simulink model "Demo_CooperativeDriving_cs"  (Simulink 7.6)
settings: Solver=ode5  SolverMode=SingleTasking  StartTime=0.0  StopTime=8  FixedStep=1/20  RelTol=1e-3
PreLoadFcn:
  | check_NUTS_defined
  | model_closed = 0;
  | assignin('base',['model_closed_' bdroot],false);
InitFcn:
  | PreScanExperimentInitFcn(bdroot)
StopFcn:
  | PreScanExperimentStopFcn(bdroot);
  | 
values from neighbouring files (symbols this model uses):
  Cf = (MLV+MRV)*g/2    (= 5460.246)    [shared_pars.m]
  Cr = (MLA+MRA)*g/2    (= 3937.734)    [shared_pars.m]
  Jzz = J_zz + 2*m_wheel*lva^2 + 2*m_wheel*laa^2    (= 3255.36268364)    [shared_pars.m]
  Kaa = 200000    [shared_pars.m]
  Kf = Kva/(g*(MLV+MRV))    (= 18.3141931701)    [shared_pars.m]
  Kr = Kaa/(g*(MLA+MRA))    (= 25.3953161895)    [shared_pars.m]
  Kva = 200000    [shared_pars.m]
  laa = l - lva    (= 1.67328601253)    [shared_pars.m]
  lva = l*(MLA+MRA)/m    (= 1.20671398747)    [shared_pars.m]
  m = MLV+MRV+MLA+MRA    (= 1916)    [shared_pars.m]
  Mu = 1    [simulinkmodel.m]
  relax_on = 0    [simulinkmodel.m]
  sigma_f = 0.65    [simulinkmodel.m]
  sigma_r = 0.65    [simulinkmodel.m]
  TyreType = 1    [simulinkmodel.m]
undefined symbols (not defined in the file or in its folder): DiscIntNeverNeededParam
libraries: PreScanSimulinkLibrary x14, PreScanUsefulBlocks x6, simulink_extras x5
(part 4 of 6)

== system Demo_CooperativeDriving_cs/Citroen_C3_1/Swarm Behavior/Polar2Cart1 ==
  R : Inport
  theta : Inport  Port=2
  Degrees to Radians : simulink_extras/Transformations/Degrees to Radians  SystemSampleTime=-1
  Fcn : Fcn  Expr=cos(-u)
  Fcn1 : Fcn  Expr=sin(-u)
  Product : Product  RndMeth=Zero
  Product1 : Product  RndMeth=Zero
  x : Outport
  y : Outport  Port=2
  wires:
  Product1/1 -> y/1
  Fcn1/1 -> Product1/2
  Product/1 -> x/1
  R/1 -> Product1/1, Product/1
  Fcn/1 -> Product/2
  Degrees to Radians/1 -> Fcn1/1, Fcn/1
  theta/1 -> Degrees to Radians/1

== system Demo_CooperativeDriving_cs/Citroen_C3_1/Swarm Behavior/Vehicle Dynamics ==
  speed : Inport
  delta : Inport  Port=2
  Mux1 : Mux  Inputs={2,1,1,2,3,3,2}
  Saturation : Saturate  UpperLimit=inf  LowerLimit=1
  Terminator22 : Terminator
  eq_of_motion : Subsystem
  slip_angles : Subsystem
  tyre_forces : Subsystem
  x_y_rotz : Outport
  wires:
  Mux1/1 -> Terminator22/1  "con_o"
  speed/1 -> Saturation/1
  eq_of_motion/3(ddy_ddpsi) -> Mux1/7  "ddy_ddpsi"
  eq_of_motion/1(x_y_psi) -> x_y_rotz/1, Mux1/5  "x_y_psi"
  tyre_forces/1(Fy_wheels) -> Mux1/1  "Fy_wheels"
  tyre_forces/2(F_lat) -> eq_of_motion/2(F_lat), Mux1/2  "Flat"
  tyre_forces/3(Mz) -> eq_of_motion/3(Mz), Mux1/3  "Mz"
  slip_angles/1(alpha) -> Mux1/4, tyre_forces/1(alpha)  "alpha"
  delta/1 -> slip_angles/2(delta), tyre_forces/2(delta)
  eq_of_motion/2(dx_dy_dpsi) -> Mux1/6, slip_angles/1(dx_dy_dpsi)  "dx_dy_dpsi"
  Saturation/1 -> eq_of_motion/1(Vx)

== system Demo_CooperativeDriving_cs/Citroen_C3_1/Swarm Behavior/xyalpha_2_state ==
  xyyaw : Inport
  Constant : Constant  Value=0
  Demux : Demux  Outputs=3
  Derivative : Derivative
  Derivative1 : Derivative
  Mux : Mux  Inputs=9
  state : Outport
  wires:
  Demux/1 -> Mux/1, Derivative/1  "x"
  Demux/2 -> Mux/2, Derivative1/1  "y"
  Constant/1 -> Mux/8, Mux/6, Mux/3, Mux/7
  xyyaw/1 -> Demux/1
  Mux/1 -> state/1
  Derivative/1 -> Mux/4
  Derivative1/1 -> Mux/5
  Demux/3 -> Mux/9  "yaw"

== system Demo_CooperativeDriving_cs/Mazda_RX8_1/SELF_Demux/compas converter ==
  rotz [rad] : Inport
  cart2compas : Subsystem
  rad2deg : Gain  Gain=180/pi
  heading [deg] : Outport
  wires:
  cart2compas/1(heading [deg]) -> heading [deg]/1
  rotz [rad]/1 -> rad2deg/1
  rad2deg/1 -> cart2compas/1(Angle [deg])

== system Demo_CooperativeDriving_cs/Mazda_RX8_1/Trajectories/Linked_to_Trajectory_1 ==
  From Workspace : FromWorkspace  VariableName=trajectory  SampleTime=TimeStep  OutputAfterFinalValue=Holding final value
  From Workspace1 : FromWorkspace  VariableName=trajectory  SampleTime=TimeStep  OutputAfterFinalValue=Setting to zero
  Mux : Mux  Inputs=2
  Selector1 : Selector  InputPortWidth=24  IndexOptions=Index vector (dialog)  Indices=[7:18]  OutputSizes=1
  Selector9 : Selector  InputPortWidth=24  IndexOptions=Index vector (dialog)  Indices=[1:6]  OutputSizes=1
  trajectory : Outport
  wires:
  Selector1/1 -> Mux/2
  Selector9/1 -> Mux/1
  Mux/1 -> trajectory/1
  From Workspace1/1 -> Selector1/1
  From Workspace/1 -> Selector9/1

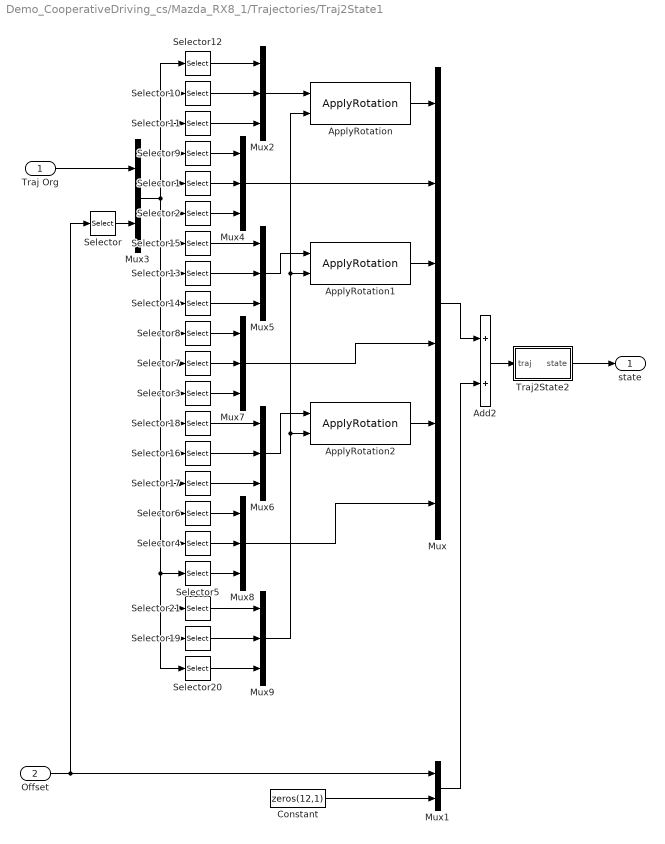
== system Demo_CooperativeDriving_cs/Mazda_RX8_1/Trajectories/Traj2State1 ==
  Traj Org : Inport
  Offset : Inport  Port=2
  Add2 : Sum
  ApplyRotation : PreScanSimulinkLibrary/ApplyRotation  SystemSampleTime=-1
  ApplyRotation1 : PreScanSimulinkLibrary/ApplyRotation  SystemSampleTime=-1
  ApplyRotation2 : PreScanSimulinkLibrary/ApplyRotation  SystemSampleTime=-1
  Constant : Constant  Value=zeros(12,1)
  Mux : Mux  Inputs=6
  Mux1 : Mux  Inputs=2
  Mux{2,4..9} (7 alike) : Mux  Inputs=3
  Mux3 : Mux  Inputs=2
  Selector : Selector  InputPortWidth=6  IndexOptions=Index vector (dialog)  Indices=[4 5 6]  OutputSizes=1
  Selector1 : Selector  InputPortWidth=21  IndexOptions=Index vector (dialog)  Indices=[5]  OutputSizes=1
  Selector10 : Selector  InputPortWidth=21  IndexOptions=Index vector (dialog)  Indices=[2]  OutputSizes=1
  Selector11 : Selector  InputPortWidth=21  IndexOptions=Index vector (dialog)  Indices=[3]  OutputSizes=1
  Selector12 : Selector  InputPortWidth=21  IndexOptions=Index vector (dialog)  Indices=[1]  OutputSizes=1
  Selector13 : Selector  InputPortWidth=21  IndexOptions=Index vector (dialog)  Indices=[8]  OutputSizes=1
  Selector14 : Selector  InputPortWidth=21  IndexOptions=Index vector (dialog)  Indices=[9]  OutputSizes=1
  Selector15 : Selector  InputPortWidth=21  IndexOptions=Index vector (dialog)  Indices=[7]  OutputSizes=1
  Selector16 : Selector  InputPortWidth=21  IndexOptions=Index vector (dialog)  Indices=[14]  OutputSizes=1
  Selector17 : Selector  InputPortWidth=21  IndexOptions=Index vector (dialog)  Indices=[15]  OutputSizes=1
  Selector18 : Selector  InputPortWidth=21  IndexOptions=Index vector (dialog)  Indices=[13]  OutputSizes=1
  Selector19 : Selector  InputPortWidth=21  IndexOptions=Index vector (dialog)  Indices=[20]  OutputSizes=1
  Selector2 : Selector  InputPortWidth=21  IndexOptions=Index vector (dialog)  Indices=[6]  OutputSizes=1
  Selector20 : Selector  InputPortWidth=21  IndexOptions=Index vector (dialog)  Indices=[21]  OutputSizes=1
  Selector21 : Selector  InputPortWidth=21  IndexOptions=Index vector (dialog)  Indices=[19]  OutputSizes=1
  Selector3 : Selector  InputPortWidth=21  IndexOptions=Index vector (dialog)  Indices=[12]  OutputSizes=1
  Selector4 : Selector  InputPortWidth=21  IndexOptions=Index vector (dialog)  Indices=[17]  OutputSizes=1
  Selector5 : Selector  InputPortWidth=21  IndexOptions=Index vector (dialog)  Indices=[18]  OutputSizes=1
  Selector6 : Selector  InputPortWidth=21  IndexOptions=Index vector (dialog)  Indices=[16]  OutputSizes=1
  Selector7 : Selector  InputPortWidth=21  IndexOptions=Index vector (dialog)  Indices=[11]  OutputSizes=1
  Selector8 : Selector  InputPortWidth=21  IndexOptions=Index vector (dialog)  Indices=[10]  OutputSizes=1
  Selector9 : Selector  InputPortWidth=21  IndexOptions=Index vector (dialog)  Indices=[4]  OutputSizes=1
  Traj2State2 : Subsystem
  state : Outport
  wires:
  Mux9/1 -> ApplyRotation2/2, ApplyRotation1/2, ApplyRotation/2
  Selector20/1 -> Mux9/3
  Selector19/1 -> Mux9/2
  Selector21/1 -> Mux9/1
  Selector5/1 -> Mux8/3
  Selector4/1 -> Mux8/2
  Selector6/1 -> Mux8/1
  Mux8/1 -> Mux/6
  Mux6/1 -> ApplyRotation2/1
  Mux7/1 -> Mux/4
  ApplyRotation2/1 -> Mux/5
  Selector3/1 -> Mux7/3
  Selector7/1 -> Mux7/2
  Selector8/1 -> Mux7/1
  Mux4/1 -> Mux/2
  Mux5/1 -> ApplyRotation1/1
  ApplyRotation1/1 -> Mux/3
  Mux2/1 -> ApplyRotation/1
  ApplyRotation/1 -> Mux/1
  Selector2/1 -> Mux4/3
  Selector1/1 -> Mux4/2
  Selector9/1 -> Mux4/1
  Selector17/1 -> Mux6/3
  Selector16/1 -> Mux6/2
  Selector18/1 -> Mux6/1
  Selector14/1 -> Mux5/3
  Selector13/1 -> Mux5/2
  Selector15/1 -> Mux5/1
  Selector11/1 -> Mux2/3
  Selector10/1 -> Mux2/2
  Selector12/1 -> Mux2/1
  Mux3/1 -> Selector8/1, Selector7/1, Selector3/1, Selector18/1, Selector16/1, Selector17/1, Selector6/1, Selector20/1, Selector19/1, Selector21/1, Selector5/1, Selector4/1, Selector14/1, Selector13/1, Selector15/1, Selector2/1, Selector1/1, Selector9/1, Selector12/1, Selector10/1, Selector11/1
  Mux1/1 -> Add2/2
  Constant/1 -> Mux1/2
  Add2/1 -> Traj2State2/1(traj)
  Selector/1 -> Mux3/2
  Traj Org/1 -> Mux3/1
  Offset/1 -> Mux1/1, Selector/1
  Mux/1 -> Add2/1
  Traj2State2/1(state) -> state/1

== system Demo_CooperativeDriving_cs/Nissan_Cabstar_1/AIR_4_Demux/Activate_Switch ==
  BeamID : Inport
  Heading : Inport  Port=2
  Constant : Constant  Value=0
  Product1 : Product  RndMeth=Zero
  Relational Operator : RelationalOperator  Operator=~=  OutDataTypeStr=boolean
  On/Off : Outport
  wires:
  Constant/1 -> Relational Operator/1
  Relational Operator/1 -> Product1/1
  BeamID/1 -> Relational Operator/2
  Product1/1 -> On/Off/1
  Heading/1 -> Product1/2

== system Demo_CooperativeDriving_cs/Nissan_Cabstar_1/AIR_4_Demux/Signal2ArrayOfSignals1 ==
  note: Set mask parameter VECTORLENGTH
      |  to MAXMESSAGES
  note: Initial state of Previous vector block
      | set to zeros(VECTORLENGTH,1)
  LoopIndex : Inport
  Element : Inport  Port=2
  Assignment : Assignment  IndexOptions=Index vector (port)  Indices=1  OutputSizes=1
  Previous vector : Memory  X0=zeros(VECTORLENGTH,1)  InheritSampleTime=on
  ArrayofElements : Outport
  wires:
  Element/1 -> Assignment/2
  LoopIndex/1 -> Assignment/3
  Previous vector/1 -> Assignment/1
  Assignment/1 -> ArrayofElements/1, Previous vector/1

== system Demo_CooperativeDriving_cs/Nissan_Cabstar_1/AIR_4_Demux/Signal2ArrayOfSignals2 ==
  note: Set mask parameter VECTORLENGTH
      |  to MAXMESSAGES
  note: Initial state of Previous vector block
      | set to zeros(VECTORLENGTH,1)
  LoopIndex : Inport
  Element : Inport  Port=2
  Assignment : Assignment  IndexOptions=Index vector (port)  Indices=1  OutputSizes=1
  Previous vector : Memory  X0=zeros(VECTORLENGTH,1)  InheritSampleTime=on
  ArrayofElements : Outport
  wires:
  Element/1 -> Assignment/2
  LoopIndex/1 -> Assignment/3
  Previous vector/1 -> Assignment/1
  Assignment/1 -> ArrayofElements/1, Previous vector/1

== system Demo_CooperativeDriving_cs/Nissan_Cabstar_1/AIR_4_Demux/Signal2ArrayOfSignals3 ==
  note: Set mask parameter VECTORLENGTH
      |  to MAXMESSAGES
  note: Initial state of Previous vector block
      | set to zeros(VECTORLENGTH,1)
  LoopIndex : Inport
  Element : Inport  Port=2
  Assignment : Assignment  IndexOptions=Index vector (port)  Indices=1  OutputSizes=1
  Previous vector : Memory  X0=zeros(VECTORLENGTH,1)  InheritSampleTime=on
  ArrayofElements : Outport
  wires:
  Element/1 -> Assignment/2
  LoopIndex/1 -> Assignment/3
  Previous vector/1 -> Assignment/1
  Assignment/1 -> ArrayofElements/1, Previous vector/1

== system Demo_CooperativeDriving_cs/Nissan_Cabstar_1/AIR_4_Demux/Signal2ArrayOfSignals4 ==
  note: Set mask parameter VECTORLENGTH
      |  to MAXMESSAGES
  note: Initial state of Previous vector block
      | set to zeros(VECTORLENGTH,1)
  LoopIndex : Inport
  Element : Inport  Port=2
  Assignment : Assignment  IndexOptions=Index vector (port)  Indices=1  OutputSizes=1
  Previous vector : Memory  X0=zeros(VECTORLENGTH,1)  InheritSampleTime=on
  ArrayofElements : Outport
  wires:
  Element/1 -> Assignment/2
  LoopIndex/1 -> Assignment/3
  Previous vector/1 -> Assignment/1
  Assignment/1 -> ArrayofElements/1, Previous vector/1

== system Demo_CooperativeDriving_cs/Nissan_Cabstar_1/AIR_4_Demux/Signal2ArrayOfSignals5 ==
  note: Set mask parameter VECTORLENGTH
      |  to MAXMESSAGES
  note: Initial state of Previous vector block
      | set to zeros(VECTORLENGTH,1)
  LoopIndex : Inport
  Element : Inport  Port=2
  Assignment : Assignment  IndexOptions=Index vector (port)  Indices=1  OutputSizes=1
  Previous vector : Memory  X0=zeros(VECTORLENGTH,1)  InheritSampleTime=on
  ArrayofElements : Outport
  wires:
  Element/1 -> Assignment/2
  LoopIndex/1 -> Assignment/3
  Previous vector/1 -> Assignment/1
  Assignment/1 -> ArrayofElements/1, Previous vector/1

== system Demo_CooperativeDriving_cs/Nissan_Cabstar_1/AIR_4_Demux/Signal2ArrayOfSignals6 ==
  note: Set mask parameter VECTORLENGTH
      |  to MAXMESSAGES
  note: Initial state of Previous vector block
      | set to zeros(VECTORLENGTH,1)
  LoopIndex : Inport
  Element : Inport  Port=2
  Assignment : Assignment  IndexOptions=Index vector (port)  Indices=1  OutputSizes=1
  Previous vector : Memory  X0=zeros(VECTORLENGTH,1)  InheritSampleTime=on
  ArrayofElements : Outport
  wires:
  Element/1 -> Assignment/2
  LoopIndex/1 -> Assignment/3
  Previous vector/1 -> Assignment/1
  Assignment/1 -> ArrayofElements/1, Previous vector/1

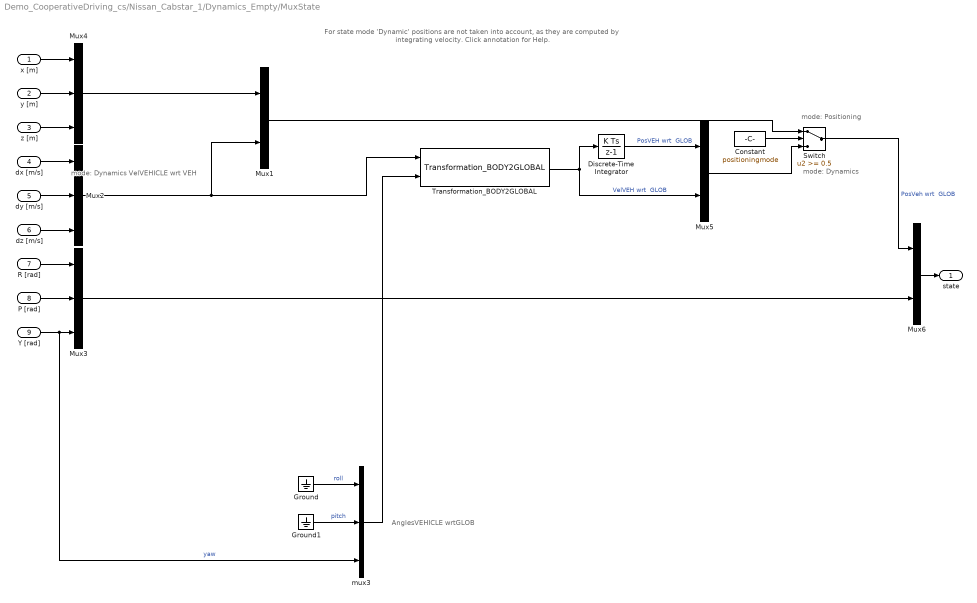
== system Demo_CooperativeDriving_cs/Nissan_Cabstar_1/Dynamics_Empty/MuxState ==
  note: mode: Dynamics
  note: mode: Positioning
  note: mode: Dynamics
      | VelVEHICLE
      | wrt VEH
  note: AnglesVEHICLE
      | wrtGLOB
  note: For state mode 'Dynamic' positions
      | are not taken into account, as they
      | are computed by integrating velocity.
      | Click annotation for Help.
  x [m] : Inport  SampleTime=TimeStep
  y [m] : Inport  Port=2  SampleTime=TimeStep
  z [m] : Inport  Port=3  SampleTime=TimeStep
  dx [m/s] : Inport  Port=4  SampleTime=TimeStep
  dy [m/s] : Inport  Port=5  SampleTime=TimeStep
  dz [m/s] : Inport  Port=6  SampleTime=TimeStep
  R [rad] : Inport  Port=7  SampleTime=TimeStep
  P [rad] : Inport  Port=8  SampleTime=TimeStep
  Y [rad] : Inport  Port=9  SampleTime=TimeStep
  Constant : Constant  DisableCoverage=on  Value=positioningmode
  Discrete-Time Integrator : DiscreteIntegrator  SampleTime=TimeStep  ICPrevOutput=DiscIntNeverNeededParam  ICPrevScaledInput=DiscIntNeverNeededParam
  Ground : Ground
  Ground1 : Ground
  Mux1 : Mux  Inputs=[3 3]
  Mux2 : Mux  Inputs=3
  Mux3 : Mux  Inputs=3
  Mux4 : Mux  Inputs=3
  Mux5 : Mux  Inputs=[3 3]
  Mux6 : Mux  Inputs=[6 3]
  Switch : Switch  Threshold=0.5
  Transformation_BODY2GLOBAL : PreScanSimulinkLibrary/Simple_Vehicle_Dynamics/Chassis/MuxDynState/Transformation_BODY2GLOBAL  SystemSampleTime=-1
  mux3 : Mux  Inputs=3
  state : Outport
  wires:
  Constant/1 -> Switch/2
  Mux6/1 -> state/1
  Mux4/1 -> Mux1/1
  Mux5/1 -> Switch/3
  Mux1/1 -> Switch/1
  Switch/1 -> Mux6/1  "PosVeh wrt  GLOB"
  P [rad]/1 -> Mux3/2
  R [rad]/1 -> Mux3/1
  dz [m/s]/1 -> Mux2/3
  dy [m/s]/1 -> Mux2/2
  dx [m/s]/1 -> Mux2/1
  z [m]/1 -> Mux4/3
  y [m]/1 -> Mux4/2
  x [m]/1 -> Mux4/1
  Ground1/1 -> mux3/2  "pitch"
  Y [rad]/1 -> mux3/3, Mux3/3  "yaw"
  Mux3/1 -> Mux6/2
  Transformation_BODY2GLOBAL/1 -> Discrete-Time Integrator/1, Mux5/2  "VelVEH wrt  GLOB"
  mux3/1 -> Transformation_BODY2GLOBAL/2
  Ground/1 -> mux3/1  "roll"
  Mux2/1 -> Mux1/2, Transformation_BODY2GLOBAL/1
  Discrete-Time Integrator/1 -> Mux5/1  "PosVEH wrt  GLOB"

== system Demo_CooperativeDriving_cs/Nissan_Cabstar_1/SELF_Demux/compas converter ==
  rotz [rad] : Inport
  cart2compas : Subsystem
  rad2deg : Gain  Gain=180/pi
  heading [deg] : Outport
  wires:
  cart2compas/1(heading [deg]) -> heading [deg]/1
  rotz [rad]/1 -> rad2deg/1
  rad2deg/1 -> cart2compas/1(Angle [deg])

== system Demo_CooperativeDriving_cs/Nissan_Cabstar_1/Swarm Behavior/Control ==
  xrel : Inport
  yrel : Inport  Port=2
  x_dist : Inport  Port=3
  y_dist : Inport  Port=4
  Add : Sum  Inputs=+-
  Add1 : Sum  Inputs=+-
  Add2 : Sum
  Complex to Magnitude-Angle1 : ComplexToMagnitudeAngle
  Gain1 : Gain  Gain=0.5  SaturateOnIntegerOverflow=on  OutDataTypeStr=Inherit: Same as input  ParamDataTypeStr=Inherit: Same as input
  Gain2 : Gain  SaturateOnIntegerOverflow=on  OutDataTypeStr=Inherit: Same as input  ParamDataTypeStr=Inherit: Same as input
  Rate Limiter : RateLimiter  SampleTimeMode=inherited
  Real-Imag to Complex1 : RealImagToComplex
  Saturation : Saturate  UpperLimit=10/180*pi  LowerLimit=-10/180*pi
  Saturation1 : Saturate  UpperLimit=200/3.6  LowerLimit=1
  Saturation2 : Saturate  UpperLimit=inf  LowerLimit=0
  Terminator_1 : Terminator
  Transfer Fcn : TransferFcn  Denominator=[0.4 1]
  preview_distance : Constant  Value=2
  v0 : Constant  Value=10
  speed : Outport
  delta : Outport  Port=2
  wires:
  Complex to Magnitude-Angle1/2 -> Gain2/1
  Add2/1 -> Rate Limiter/1
  v0/1 -> Add2/2
  Gain1/1 -> Add2/1
  Real-Imag to Complex1/1 -> Complex to Magnitude-Angle1/1
  Add/1 -> Transfer Fcn/1
  y_dist/1 -> Add1/2
  x_dist/1 -> Saturation2/1
  Add1/1 -> Real-Imag to Complex1/2
  Transfer Fcn/1 -> Gain1/1
  yrel/1 -> Add1/1
  xrel/1 -> Add/1
  preview_distance/1 -> Real-Imag to Complex1/1
  Saturation/1 -> delta/1
  Saturation1/1 -> speed/1
  Rate Limiter/1 -> Saturation1/1
  Saturation2/1 -> Add/2
  Gain2/1 -> Saturation/1
  Complex to Magnitude-Angle1/1 -> Terminator_1/1

== system Demo_CooperativeDriving_cs/Nissan_Cabstar_1/Swarm Behavior/Master_detector ==
  id : Inport
  "Range " : Inport  Port=2
  "theta " : Inport  Port=3
  ids : Inport  Port=4
  Product : Product  RndMeth=Zero
  Product1 : Product  RndMeth=Zero
  Relational Operator : RelationalOperator  Operator===  OutDataTypeStr=boolean  InputSameDT=on
  Sum of Elements : Sum  Inputs=+
  Sum of Elements1 : Sum  Inputs=+
  Range : Outport
  theta : Outport  Port=2
  wires:
  Product1/1 -> Sum of Elements1/1
  Sum of Elements1/1 -> theta/1
  "theta "/1 -> Product1/2
  Sum of Elements/1 -> Range/1
  "Range "/1 -> Product/2
  id/1 -> Relational Operator/2
  ids/1 -> Relational Operator/1
  Product/1 -> Sum of Elements/1
  Relational Operator/1 -> Product/1, Product1/1

== system Demo_CooperativeDriving_cs/Nissan_Cabstar_1/Swarm Behavior/Polar2Cart1 ==
  R : Inport
  theta : Inport  Port=2
  Degrees to Radians : simulink_extras/Transformations/Degrees to Radians  SystemSampleTime=-1
  Fcn : Fcn  Expr=cos(-u)
  Fcn1 : Fcn  Expr=sin(-u)
  Product : Product  RndMeth=Zero
  Product1 : Product  RndMeth=Zero
  x : Outport
  y : Outport  Port=2
  wires:
  Product1/1 -> y/1
  Fcn1/1 -> Product1/2
  Product/1 -> x/1
  R/1 -> Product1/1, Product/1
  Fcn/1 -> Product/2
  Degrees to Radians/1 -> Fcn1/1, Fcn/1
  theta/1 -> Degrees to Radians/1

== system Demo_CooperativeDriving_cs/Nissan_Cabstar_1/Swarm Behavior/Vehicle Dynamics ==
  speed : Inport
  delta : Inport  Port=2
  Mux1 : Mux  Inputs={2,1,1,2,3,3,2}
  Saturation : Saturate  UpperLimit=inf  LowerLimit=1
  Terminator22 : Terminator
  eq_of_motion : Subsystem
  slip_angles : Subsystem
  tyre_forces : Subsystem
  x_y_rotz : Outport
  wires:
  Mux1/1 -> Terminator22/1  "con_o"
  speed/1 -> Saturation/1
  eq_of_motion/3(ddy_ddpsi) -> Mux1/7  "ddy_ddpsi"
  eq_of_motion/1(x_y_psi) -> x_y_rotz/1, Mux1/5  "x_y_psi"
  tyre_forces/1(Fy_wheels) -> Mux1/1  "Fy_wheels"
  tyre_forces/2(F_lat) -> eq_of_motion/2(F_lat), Mux1/2  "Flat"
  tyre_forces/3(Mz) -> eq_of_motion/3(Mz), Mux1/3  "Mz"
  slip_angles/1(alpha) -> Mux1/4, tyre_forces/1(alpha)  "alpha"
  delta/1 -> slip_angles/2(delta), tyre_forces/2(delta)
  eq_of_motion/2(dx_dy_dpsi) -> Mux1/6, slip_angles/1(dx_dy_dpsi)  "dx_dy_dpsi"
  Saturation/1 -> eq_of_motion/1(Vx)

== system Demo_CooperativeDriving_cs/Nissan_Cabstar_1/Swarm Behavior/xyalpha_2_state ==
  xyyaw : Inport
  Constant : Constant  Value=0
  Demux : Demux  Outputs=3
  Derivative : Derivative
  Derivative1 : Derivative
  Mux : Mux  Inputs=9
  state : Outport
  wires:
  Demux/1 -> Mux/1, Derivative/1  "x"
  Demux/2 -> Mux/2, Derivative1/1  "y"
  Constant/1 -> Mux/8, Mux/6, Mux/3, Mux/7
  xyyaw/1 -> Demux/1
  Mux/1 -> state/1
  Derivative/1 -> Mux/4
  Derivative1/1 -> Mux/5
  Demux/3 -> Mux/9  "yaw"

== system Demo_CooperativeDriving_cs/Toyota_Previa_1/AIR_1_Demux/Activate_Switch ==
  BeamID : Inport
  Heading : Inport  Port=2
  Constant : Constant  Value=0
  Product1 : Product  RndMeth=Zero
  Relational Operator : RelationalOperator  Operator=~=  OutDataTypeStr=boolean
  On/Off : Outport
  wires:
  Constant/1 -> Relational Operator/1
  Relational Operator/1 -> Product1/1
  BeamID/1 -> Relational Operator/2
  Product1/1 -> On/Off/1
  Heading/1 -> Product1/2

== system Demo_CooperativeDriving_cs/Toyota_Previa_1/AIR_1_Demux/Signal2ArrayOfSignals1 ==
  note: Set mask parameter VECTORLENGTH
      |  to MAXMESSAGES
  note: Initial state of Previous vector block
      | set to zeros(VECTORLENGTH,1)
  LoopIndex : Inport
  Element : Inport  Port=2
  Assignment : Assignment  IndexOptions=Index vector (port)  Indices=1  OutputSizes=1
  Previous vector : Memory  X0=zeros(VECTORLENGTH,1)  InheritSampleTime=on
  ArrayofElements : Outport
  wires:
  Element/1 -> Assignment/2
  LoopIndex/1 -> Assignment/3
  Previous vector/1 -> Assignment/1
  Assignment/1 -> ArrayofElements/1, Previous vector/1

== system Demo_CooperativeDriving_cs/Toyota_Previa_1/AIR_1_Demux/Signal2ArrayOfSignals2 ==
  note: Set mask parameter VECTORLENGTH
      |  to MAXMESSAGES
  note: Initial state of Previous vector block
      | set to zeros(VECTORLENGTH,1)
  LoopIndex : Inport
  Element : Inport  Port=2
  Assignment : Assignment  IndexOptions=Index vector (port)  Indices=1  OutputSizes=1
  Previous vector : Memory  X0=zeros(VECTORLENGTH,1)  InheritSampleTime=on
  ArrayofElements : Outport
  wires:
  Element/1 -> Assignment/2
  LoopIndex/1 -> Assignment/3
  Previous vector/1 -> Assignment/1
  Assignment/1 -> ArrayofElements/1, Previous vector/1

== system Demo_CooperativeDriving_cs/Toyota_Previa_1/AIR_1_Demux/Signal2ArrayOfSignals3 ==
  note: Set mask parameter VECTORLENGTH
      |  to MAXMESSAGES
  note: Initial state of Previous vector block
      | set to zeros(VECTORLENGTH,1)
  LoopIndex : Inport
  Element : Inport  Port=2
  Assignment : Assignment  IndexOptions=Index vector (port)  Indices=1  OutputSizes=1
  Previous vector : Memory  X0=zeros(VECTORLENGTH,1)  InheritSampleTime=on
  ArrayofElements : Outport
  wires:
  Element/1 -> Assignment/2
  LoopIndex/1 -> Assignment/3
  Previous vector/1 -> Assignment/1
  Assignment/1 -> ArrayofElements/1, Previous vector/1

== system Demo_CooperativeDriving_cs/Toyota_Previa_1/AIR_1_Demux/Signal2ArrayOfSignals4 ==
  note: Set mask parameter VECTORLENGTH
      |  to MAXMESSAGES
  note: Initial state of Previous vector block
      | set to zeros(VECTORLENGTH,1)
  LoopIndex : Inport
  Element : Inport  Port=2
  Assignment : Assignment  IndexOptions=Index vector (port)  Indices=1  OutputSizes=1
  Previous vector : Memory  X0=zeros(VECTORLENGTH,1)  InheritSampleTime=on
  ArrayofElements : Outport
  wires:
  Element/1 -> Assignment/2
  LoopIndex/1 -> Assignment/3
  Previous vector/1 -> Assignment/1
  Assignment/1 -> ArrayofElements/1, Previous vector/1

== system Demo_CooperativeDriving_cs/Toyota_Previa_1/AIR_1_Demux/Signal2ArrayOfSignals5 ==
  note: Set mask parameter VECTORLENGTH
      |  to MAXMESSAGES
  note: Initial state of Previous vector block
      | set to zeros(VECTORLENGTH,1)
  LoopIndex : Inport
  Element : Inport  Port=2
  Assignment : Assignment  IndexOptions=Index vector (port)  Indices=1  OutputSizes=1
  Previous vector : Memory  X0=zeros(VECTORLENGTH,1)  InheritSampleTime=on
  ArrayofElements : Outport
  wires:
  Element/1 -> Assignment/2
  LoopIndex/1 -> Assignment/3
  Previous vector/1 -> Assignment/1
  Assignment/1 -> ArrayofElements/1, Previous vector/1

== system Demo_CooperativeDriving_cs/Toyota_Previa_1/AIR_1_Demux/Signal2ArrayOfSignals6 ==
  note: Set mask parameter VECTORLENGTH
      |  to MAXMESSAGES
  note: Initial state of Previous vector block
      | set to zeros(VECTORLENGTH,1)
  LoopIndex : Inport
  Element : Inport  Port=2
  Assignment : Assignment  IndexOptions=Index vector (port)  Indices=1  OutputSizes=1
  Previous vector : Memory  X0=zeros(VECTORLENGTH,1)  InheritSampleTime=on
  ArrayofElements : Outport
  wires:
  Element/1 -> Assignment/2
  LoopIndex/1 -> Assignment/3
  Previous vector/1 -> Assignment/1
  Assignment/1 -> ArrayofElements/1, Previous vector/1

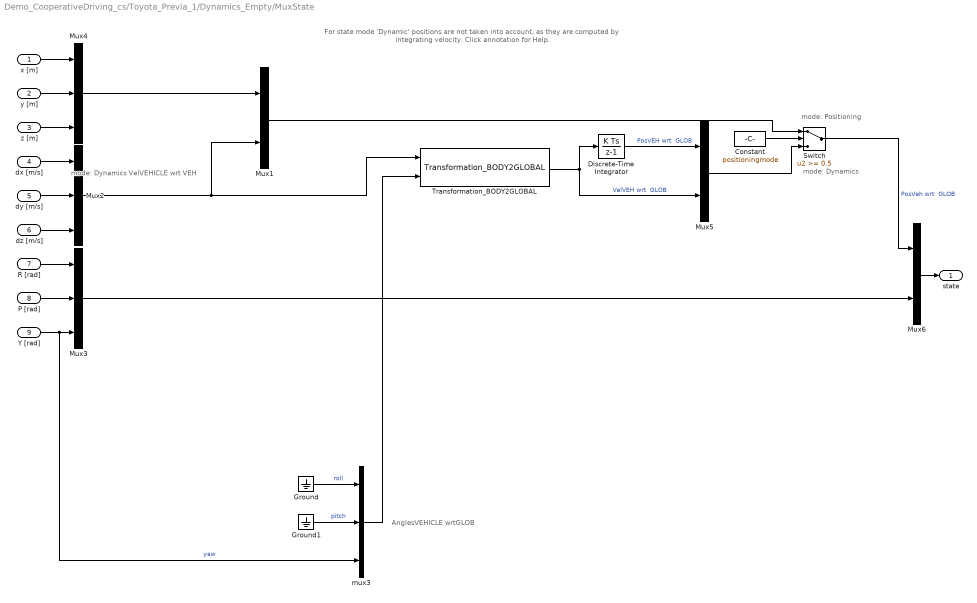
== system Demo_CooperativeDriving_cs/Toyota_Previa_1/Dynamics_Empty/MuxState ==
  note: mode: Dynamics
  note: mode: Positioning
  note: mode: Dynamics
      | VelVEHICLE
      | wrt VEH
  note: AnglesVEHICLE
      | wrtGLOB
  note: For state mode 'Dynamic' positions
      | are not taken into account, as they
      | are computed by integrating velocity.
      | Click annotation for Help.
  x [m] : Inport  SampleTime=TimeStep
  y [m] : Inport  Port=2  SampleTime=TimeStep
  z [m] : Inport  Port=3  SampleTime=TimeStep
  dx [m/s] : Inport  Port=4  SampleTime=TimeStep
  dy [m/s] : Inport  Port=5  SampleTime=TimeStep
  dz [m/s] : Inport  Port=6  SampleTime=TimeStep
  R [rad] : Inport  Port=7  SampleTime=TimeStep
  P [rad] : Inport  Port=8  SampleTime=TimeStep
  Y [rad] : Inport  Port=9  SampleTime=TimeStep
  Constant : Constant  DisableCoverage=on  Value=positioningmode
  Discrete-Time Integrator : DiscreteIntegrator  SampleTime=TimeStep  ICPrevOutput=DiscIntNeverNeededParam  ICPrevScaledInput=DiscIntNeverNeededParam
  Ground : Ground
  Ground1 : Ground
  Mux1 : Mux  Inputs=[3 3]
  Mux2 : Mux  Inputs=3
  Mux3 : Mux  Inputs=3
  Mux4 : Mux  Inputs=3
  Mux5 : Mux  Inputs=[3 3]
  Mux6 : Mux  Inputs=[6 3]
  Switch : Switch  Threshold=0.5
  Transformation_BODY2GLOBAL : PreScanSimulinkLibrary/Simple_Vehicle_Dynamics/Chassis/MuxDynState/Transformation_BODY2GLOBAL  SystemSampleTime=-1
  mux3 : Mux  Inputs=3
  state : Outport
  wires:
  Constant/1 -> Switch/2
  Mux6/1 -> state/1
  Mux4/1 -> Mux1/1
  Mux5/1 -> Switch/3
  Mux1/1 -> Switch/1
  Switch/1 -> Mux6/1  "PosVeh wrt  GLOB"
  P [rad]/1 -> Mux3/2
  R [rad]/1 -> Mux3/1
  dz [m/s]/1 -> Mux2/3
  dy [m/s]/1 -> Mux2/2
  dx [m/s]/1 -> Mux2/1
  z [m]/1 -> Mux4/3
  y [m]/1 -> Mux4/2
  x [m]/1 -> Mux4/1
  Ground1/1 -> mux3/2  "pitch"
  Y [rad]/1 -> mux3/3, Mux3/3  "yaw"
  Mux3/1 -> Mux6/2
  Transformation_BODY2GLOBAL/1 -> Discrete-Time Integrator/1, Mux5/2  "VelVEH wrt  GLOB"
  mux3/1 -> Transformation_BODY2GLOBAL/2
  Ground/1 -> mux3/1  "roll"
  Mux2/1 -> Mux1/2, Transformation_BODY2GLOBAL/1
  Discrete-Time Integrator/1 -> Mux5/1  "PosVEH wrt  GLOB"

== system Demo_CooperativeDriving_cs/Toyota_Previa_1/SELF_Demux/compas converter ==
  rotz [rad] : Inport
  cart2compas : Subsystem
  rad2deg : Gain  Gain=180/pi
  heading [deg] : Outport
  wires:
  cart2compas/1(heading [deg]) -> heading [deg]/1
  rotz [rad]/1 -> rad2deg/1
  rad2deg/1 -> cart2compas/1(Angle [deg])

== system Demo_CooperativeDriving_cs/Toyota_Previa_1/Swarm Behavior/Control ==
  xrel : Inport
  yrel : Inport  Port=2
  x_dist : Inport  Port=3
  y_dist : Inport  Port=4
  Add : Sum  Inputs=+-
  Add1 : Sum  Inputs=+-
  Add2 : Sum
  Complex to Magnitude-Angle1 : ComplexToMagnitudeAngle
  Gain1 : Gain  Gain=0.5  SaturateOnIntegerOverflow=on  OutDataTypeStr=Inherit: Same as input  ParamDataTypeStr=Inherit: Same as input
  Gain2 : Gain  SaturateOnIntegerOverflow=on  OutDataTypeStr=Inherit: Same as input  ParamDataTypeStr=Inherit: Same as input
  Rate Limiter : RateLimiter  SampleTimeMode=inherited
  Real-Imag to Complex1 : RealImagToComplex
  Saturation : Saturate  UpperLimit=10/180*pi  LowerLimit=-10/180*pi
  Saturation1 : Saturate  UpperLimit=200/3.6  LowerLimit=1
  Saturation2 : Saturate  UpperLimit=inf  LowerLimit=0
  Terminator_1 : Terminator
  Transfer Fcn : TransferFcn  Denominator=[0.4 1]
  preview_distance : Constant  Value=2
  v0 : Constant  Value=10
  speed : Outport
  delta : Outport  Port=2
  wires:
  Complex to Magnitude-Angle1/2 -> Gain2/1
  Add2/1 -> Rate Limiter/1
  v0/1 -> Add2/2
  Gain1/1 -> Add2/1
  Real-Imag to Complex1/1 -> Complex to Magnitude-Angle1/1
  Add/1 -> Transfer Fcn/1
  y_dist/1 -> Add1/2
  x_dist/1 -> Saturation2/1
  Add1/1 -> Real-Imag to Complex1/2
  Transfer Fcn/1 -> Gain1/1
  yrel/1 -> Add1/1
  xrel/1 -> Add/1
  preview_distance/1 -> Real-Imag to Complex1/1
  Saturation/1 -> delta/1
  Saturation1/1 -> speed/1
  Rate Limiter/1 -> Saturation1/1
  Saturation2/1 -> Add/2
  Gain2/1 -> Saturation/1
  Complex to Magnitude-Angle1/1 -> Terminator_1/1

== system Demo_CooperativeDriving_cs/Toyota_Previa_1/Swarm Behavior/Master_detector ==
  id : Inport
  "Range " : Inport  Port=2
  "theta " : Inport  Port=3
  ids : Inport  Port=4
  Product : Product  RndMeth=Zero
  Product1 : Product  RndMeth=Zero
  Relational Operator : RelationalOperator  Operator===  OutDataTypeStr=boolean  InputSameDT=on
  Sum of Elements : Sum  Inputs=+
  Sum of Elements1 : Sum  Inputs=+
  Range : Outport
  theta : Outport  Port=2
  wires:
  Product1/1 -> Sum of Elements1/1
  Sum of Elements1/1 -> theta/1
  "theta "/1 -> Product1/2
  Sum of Elements/1 -> Range/1
  "Range "/1 -> Product/2
  id/1 -> Relational Operator/2
  ids/1 -> Relational Operator/1
  Product/1 -> Sum of Elements/1
  Relational Operator/1 -> Product/1, Product1/1

== system Demo_CooperativeDriving_cs/Toyota_Previa_1/Swarm Behavior/Polar2Cart1 ==
  R : Inport
  theta : Inport  Port=2
  Degrees to Radians : simulink_extras/Transformations/Degrees to Radians  SystemSampleTime=-1
  Fcn : Fcn  Expr=cos(-u)
  Fcn1 : Fcn  Expr=sin(-u)
  Product : Product  RndMeth=Zero
  Product1 : Product  RndMeth=Zero
  x : Outport
  y : Outport  Port=2
  wires:
  Product1/1 -> y/1
  Fcn1/1 -> Product1/2
  Product/1 -> x/1
  R/1 -> Product1/1, Product/1
  Fcn/1 -> Product/2
  Degrees to Radians/1 -> Fcn1/1, Fcn/1
  theta/1 -> Degrees to Radians/1

== system Demo_CooperativeDriving_cs/Toyota_Previa_1/Swarm Behavior/Vehicle ==
  speed : Inport
  delta : Inport  Port=2
  Mux1 : Mux  Inputs={2,1,1,2,3,3,2}
  Saturation : Saturate  UpperLimit=inf  LowerLimit=1
  Terminator22 : Terminator
  eq_of_motion : Subsystem
  slip_angles : Subsystem
  tyre_forces : Subsystem
  x_y_rotz : Outport
  wires:
  Mux1/1 -> Terminator22/1  "con_o"
  speed/1 -> Saturation/1
  eq_of_motion/3(ddy_ddpsi) -> Mux1/7  "ddy_ddpsi"
  eq_of_motion/1(x_y_psi) -> x_y_rotz/1, Mux1/5  "x_y_psi"
  tyre_forces/1(Fy_wheels) -> Mux1/1  "Fy_wheels"
  tyre_forces/2(F_lat) -> eq_of_motion/2(F_lat), Mux1/2  "Flat"
  tyre_forces/3(Mz) -> eq_of_motion/3(Mz), Mux1/3  "Mz"
  slip_angles/1(alpha) -> Mux1/4, tyre_forces/1(alpha)  "alpha"
  delta/1 -> slip_angles/2(delta), tyre_forces/2(delta)
  eq_of_motion/2(dx_dy_dpsi) -> Mux1/6, slip_angles/1(dx_dy_dpsi)  "dx_dy_dpsi"
  Saturation/1 -> eq_of_motion/1(Vx)

== system Demo_CooperativeDriving_cs/Toyota_Previa_1/Swarm Behavior/xyalpha_2_state ==
  xyyaw : Inport
  Constant : Constant  Value=0
  Demux : Demux  Outputs=3
  Derivative : Derivative
  Derivative1 : Derivative
  Mux : Mux  Inputs=9
  state : Outport
  wires:
  Demux/1 -> Mux/1, Derivative/1  "x"
  Demux/2 -> Mux/2, Derivative1/1  "y"
  Constant/1 -> Mux/8, Mux/6, Mux/3, Mux/7
  xyyaw/1 -> Demux/1
  Mux/1 -> state/1
  Derivative/1 -> Mux/4
  Derivative1/1 -> Mux/5
  Demux/3 -> Mux/9  "yaw"

== system Demo_CooperativeDriving_cs/Toyota_Yaris_1/AIR_2_Demux/Activate_Switch ==
  BeamID : Inport
  Heading : Inport  Port=2
  Constant : Constant  Value=0
  Product1 : Product  RndMeth=Zero
  Relational Operator : RelationalOperator  Operator=~=  OutDataTypeStr=boolean
  On/Off : Outport
  wires:
  Constant/1 -> Relational Operator/1
  Relational Operator/1 -> Product1/1
  BeamID/1 -> Relational Operator/2
  Product1/1 -> On/Off/1
  Heading/1 -> Product1/2

== system Demo_CooperativeDriving_cs/Toyota_Yaris_1/AIR_2_Demux/Signal2ArrayOfSignals1 ==
  note: Set mask parameter VECTORLENGTH
      |  to MAXMESSAGES
  note: Initial state of Previous vector block
      | set to zeros(VECTORLENGTH,1)
  LoopIndex : Inport
  Element : Inport  Port=2
  Assignment : Assignment  IndexOptions=Index vector (port)  Indices=1  OutputSizes=1
  Previous vector : Memory  X0=zeros(VECTORLENGTH,1)  InheritSampleTime=on
  ArrayofElements : Outport
  wires:
  Element/1 -> Assignment/2
  LoopIndex/1 -> Assignment/3
  Previous vector/1 -> Assignment/1
  Assignment/1 -> ArrayofElements/1, Previous vector/1

== system Demo_CooperativeDriving_cs/Toyota_Yaris_1/AIR_2_Demux/Signal2ArrayOfSignals2 ==
  note: Set mask parameter VECTORLENGTH
      |  to MAXMESSAGES
  note: Initial state of Previous vector block
      | set to zeros(VECTORLENGTH,1)
  LoopIndex : Inport
  Element : Inport  Port=2
  Assignment : Assignment  IndexOptions=Index vector (port)  Indices=1  OutputSizes=1
  Previous vector : Memory  X0=zeros(VECTORLENGTH,1)  InheritSampleTime=on
  ArrayofElements : Outport
  wires:
  Element/1 -> Assignment/2
  LoopIndex/1 -> Assignment/3
  Previous vector/1 -> Assignment/1
  Assignment/1 -> ArrayofElements/1, Previous vector/1

== system Demo_CooperativeDriving_cs/Toyota_Yaris_1/AIR_2_Demux/Signal2ArrayOfSignals3 ==
  note: Set mask parameter VECTORLENGTH
      |  to MAXMESSAGES
  note: Initial state of Previous vector block
      | set to zeros(VECTORLENGTH,1)
  LoopIndex : Inport
  Element : Inport  Port=2
  Assignment : Assignment  IndexOptions=Index vector (port)  Indices=1  OutputSizes=1
  Previous vector : Memory  X0=zeros(VECTORLENGTH,1)  InheritSampleTime=on
  ArrayofElements : Outport
  wires:
  Element/1 -> Assignment/2
  LoopIndex/1 -> Assignment/3
  Previous vector/1 -> Assignment/1
  Assignment/1 -> ArrayofElements/1, Previous vector/1

== system Demo_CooperativeDriving_cs/Toyota_Yaris_1/AIR_2_Demux/Signal2ArrayOfSignals4 ==
  note: Set mask parameter VECTORLENGTH
      |  to MAXMESSAGES
  note: Initial state of Previous vector block
      | set to zeros(VECTORLENGTH,1)
  LoopIndex : Inport
  Element : Inport  Port=2
  Assignment : Assignment  IndexOptions=Index vector (port)  Indices=1  OutputSizes=1
  Previous vector : Memory  X0=zeros(VECTORLENGTH,1)  InheritSampleTime=on
  ArrayofElements : Outport
  wires:
  Element/1 -> Assignment/2
  LoopIndex/1 -> Assignment/3
  Previous vector/1 -> Assignment/1
  Assignment/1 -> ArrayofElements/1, Previous vector/1

== system Demo_CooperativeDriving_cs/Toyota_Yaris_1/AIR_2_Demux/Signal2ArrayOfSignals5 ==
  note: Set mask parameter VECTORLENGTH
      |  to MAXMESSAGES
  note: Initial state of Previous vector block
      | set to zeros(VECTORLENGTH,1)
  LoopIndex : Inport
  Element : Inport  Port=2
  Assignment : Assignment  IndexOptions=Index vector (port)  Indices=1  OutputSizes=1
  Previous vector : Memory  X0=zeros(VECTORLENGTH,1)  InheritSampleTime=on
  ArrayofElements : Outport
  wires:
  Element/1 -> Assignment/2
  LoopIndex/1 -> Assignment/3
  Previous vector/1 -> Assignment/1
  Assignment/1 -> ArrayofElements/1, Previous vector/1

== system Demo_CooperativeDriving_cs/Toyota_Yaris_1/AIR_2_Demux/Signal2ArrayOfSignals6 ==
  note: Set mask parameter VECTORLENGTH
      |  to MAXMESSAGES
  note: Initial state of Previous vector block
      | set to zeros(VECTORLENGTH,1)
  LoopIndex : Inport
  Element : Inport  Port=2
  Assignment : Assignment  IndexOptions=Index vector (port)  Indices=1  OutputSizes=1
  Previous vector : Memory  X0=zeros(VECTORLENGTH,1)  InheritSampleTime=on
  ArrayofElements : Outport
  wires:
  Element/1 -> Assignment/2
  LoopIndex/1 -> Assignment/3
  Previous vector/1 -> Assignment/1
  Assignment/1 -> ArrayofElements/1, Previous vector/1

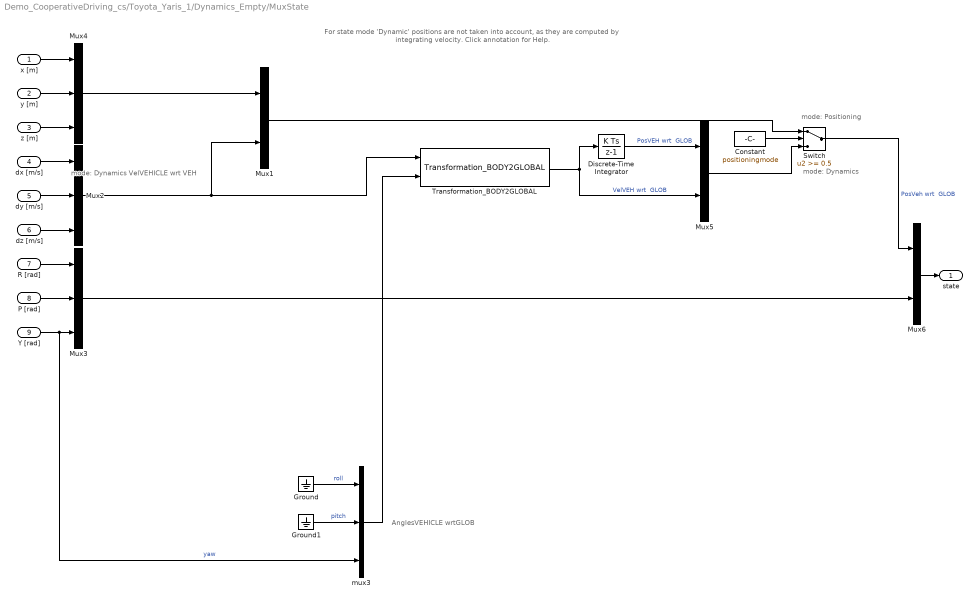
== system Demo_CooperativeDriving_cs/Toyota_Yaris_1/Dynamics_Empty/MuxState ==
  note: mode: Dynamics
  note: mode: Positioning
  note: mode: Dynamics
      | VelVEHICLE
      | wrt VEH
  note: AnglesVEHICLE
      | wrtGLOB
  note: For state mode 'Dynamic' positions
      | are not taken into account, as they
      | are computed by integrating velocity.
      | Click annotation for Help.
  x [m] : Inport  SampleTime=TimeStep
  y [m] : Inport  Port=2  SampleTime=TimeStep
  z [m] : Inport  Port=3  SampleTime=TimeStep
  dx [m/s] : Inport  Port=4  SampleTime=TimeStep
  dy [m/s] : Inport  Port=5  SampleTime=TimeStep
  dz [m/s] : Inport  Port=6  SampleTime=TimeStep
  R [rad] : Inport  Port=7  SampleTime=TimeStep
  P [rad] : Inport  Port=8  SampleTime=TimeStep
  Y [rad] : Inport  Port=9  SampleTime=TimeStep
  Constant : Constant  DisableCoverage=on  Value=positioningmode
  Discrete-Time Integrator : DiscreteIntegrator  SampleTime=TimeStep  ICPrevOutput=DiscIntNeverNeededParam  ICPrevScaledInput=DiscIntNeverNeededParam
  Ground : Ground
  Ground1 : Ground
  Mux1 : Mux  Inputs=[3 3]
  Mux2 : Mux  Inputs=3
  Mux3 : Mux  Inputs=3
  Mux4 : Mux  Inputs=3
  Mux5 : Mux  Inputs=[3 3]
  Mux6 : Mux  Inputs=[6 3]
  Switch : Switch  Threshold=0.5
  Transformation_BODY2GLOBAL : PreScanSimulinkLibrary/Simple_Vehicle_Dynamics/Chassis/MuxDynState/Transformation_BODY2GLOBAL  SystemSampleTime=-1
  mux3 : Mux  Inputs=3
  state : Outport
  wires:
  Constant/1 -> Switch/2
  Mux6/1 -> state/1
  Mux4/1 -> Mux1/1
  Mux5/1 -> Switch/3
  Mux1/1 -> Switch/1
  Switch/1 -> Mux6/1  "PosVeh wrt  GLOB"
  P [rad]/1 -> Mux3/2
  R [rad]/1 -> Mux3/1
  dz [m/s]/1 -> Mux2/3
  dy [m/s]/1 -> Mux2/2
  dx [m/s]/1 -> Mux2/1
  z [m]/1 -> Mux4/3
  y [m]/1 -> Mux4/2
  x [m]/1 -> Mux4/1
  Ground1/1 -> mux3/2  "pitch"
  Y [rad]/1 -> mux3/3, Mux3/3  "yaw"
  Mux3/1 -> Mux6/2
  Transformation_BODY2GLOBAL/1 -> Discrete-Time Integrator/1, Mux5/2  "VelVEH wrt  GLOB"
  mux3/1 -> Transformation_BODY2GLOBAL/2
  Ground/1 -> mux3/1  "roll"
  Mux2/1 -> Mux1/2, Transformation_BODY2GLOBAL/1
  Discrete-Time Integrator/1 -> Mux5/1  "PosVEH wrt  GLOB"

== system Demo_CooperativeDriving_cs/Toyota_Yaris_1/SELF_Demux/compas converter ==
  rotz [rad] : Inport
  cart2compas : Subsystem
  rad2deg : Gain  Gain=180/pi
  heading [deg] : Outport
  wires:
  cart2compas/1(heading [deg]) -> heading [deg]/1
  rotz [rad]/1 -> rad2deg/1
  rad2deg/1 -> cart2compas/1(Angle [deg])

== system Demo_CooperativeDriving_cs/Toyota_Yaris_1/Swarm Behavior/Control ==
  xrel : Inport
  yrel : Inport  Port=2
  x_dist : Inport  Port=3
  y_dist : Inport  Port=4
  Add : Sum  Inputs=+-
  Add1 : Sum  Inputs=+-
  Add2 : Sum
  Complex to Magnitude-Angle1 : ComplexToMagnitudeAngle
  Gain1 : Gain  Gain=0.5  SaturateOnIntegerOverflow=on  OutDataTypeStr=Inherit: Same as input  ParamDataTypeStr=Inherit: Same as input
  Gain2 : Gain  SaturateOnIntegerOverflow=on  OutDataTypeStr=Inherit: Same as input  ParamDataTypeStr=Inherit: Same as input
  Rate Limiter : RateLimiter  SampleTimeMode=inherited
  Real-Imag to Complex1 : RealImagToComplex
  Saturation : Saturate  UpperLimit=10/180*pi  LowerLimit=-10/180*pi
  Saturation1 : Saturate  UpperLimit=200/3.6  LowerLimit=1
  Saturation2 : Saturate  UpperLimit=inf  LowerLimit=0
  Terminator_1 : Terminator
  Transfer Fcn : TransferFcn  Denominator=[0.4 1]
  preview_distance : Constant  Value=2
  v0 : Constant  Value=10
  speed : Outport
  delta : Outport  Port=2
  wires:
  Complex to Magnitude-Angle1/2 -> Gain2/1
  Add2/1 -> Rate Limiter/1
  v0/1 -> Add2/2
  Gain1/1 -> Add2/1
  Real-Imag to Complex1/1 -> Complex to Magnitude-Angle1/1
  Add/1 -> Transfer Fcn/1
  y_dist/1 -> Add1/2
  x_dist/1 -> Saturation2/1
  Add1/1 -> Real-Imag to Complex1/2
  Transfer Fcn/1 -> Gain1/1
  yrel/1 -> Add1/1
  xrel/1 -> Add/1
  preview_distance/1 -> Real-Imag to Complex1/1
  Saturation/1 -> delta/1
  Saturation1/1 -> speed/1
  Rate Limiter/1 -> Saturation1/1
  Saturation2/1 -> Add/2
  Gain2/1 -> Saturation/1
  Complex to Magnitude-Angle1/1 -> Terminator_1/1

== system Demo_CooperativeDriving_cs/Toyota_Yaris_1/Swarm Behavior/Master_detector ==
  id : Inport
  "Range " : Inport  Port=2
  "theta " : Inport  Port=3
  ids : Inport  Port=4
  Product : Product  RndMeth=Zero
  Product1 : Product  RndMeth=Zero
  Relational Operator : RelationalOperator  Operator===  OutDataTypeStr=boolean  InputSameDT=on
  Sum of Elements : Sum  Inputs=+
  Sum of Elements1 : Sum  Inputs=+
  Range : Outport
  theta : Outport  Port=2
  wires:
  Product1/1 -> Sum of Elements1/1
  Sum of Elements1/1 -> theta/1
  "theta "/1 -> Product1/2
  Sum of Elements/1 -> Range/1
  "Range "/1 -> Product/2
  id/1 -> Relational Operator/2
  ids/1 -> Relational Operator/1
  Product/1 -> Sum of Elements/1
  Relational Operator/1 -> Product/1, Product1/1

== system Demo_CooperativeDriving_cs/Toyota_Yaris_1/Swarm Behavior/Polar2Cart1 ==
  R : Inport
  theta : Inport  Port=2
  Degrees to Radians : simulink_extras/Transformations/Degrees to Radians  SystemSampleTime=-1
  Fcn : Fcn  Expr=cos(-u)
  Fcn1 : Fcn  Expr=sin(-u)
  Product : Product  RndMeth=Zero
  Product1 : Product  RndMeth=Zero
  x : Outport
  y : Outport  Port=2
  wires:
  Product1/1 -> y/1
  Fcn1/1 -> Product1/2
  Product/1 -> x/1
  R/1 -> Product1/1, Product/1
  Fcn/1 -> Product/2
  Degrees to Radians/1 -> Fcn1/1, Fcn/1
  theta/1 -> Degrees to Radians/1

== system Demo_CooperativeDriving_cs/Toyota_Yaris_1/Swarm Behavior/Vehicle Dynamics ==
  speed : Inport
  delta : Inport  Port=2
  Mux1 : Mux  Inputs={2,1,1,2,3,3,2}
  Saturation : Saturate  UpperLimit=inf  LowerLimit=1
  Terminator22 : Terminator
  eq_of_motion : Subsystem
  slip_angles : Subsystem
  tyre_forces : Subsystem
  x_y_rotz : Outport
  wires:
  Mux1/1 -> Terminator22/1  "con_o"
  speed/1 -> Saturation/1
  eq_of_motion/3(ddy_ddpsi) -> Mux1/7  "ddy_ddpsi"
  eq_of_motion/1(x_y_psi) -> x_y_rotz/1, Mux1/5  "x_y_psi"
  tyre_forces/1(Fy_wheels) -> Mux1/1  "Fy_wheels"
  tyre_forces/2(F_lat) -> eq_of_motion/2(F_lat), Mux1/2  "Flat"
  tyre_forces/3(Mz) -> eq_of_motion/3(Mz), Mux1/3  "Mz"
  slip_angles/1(alpha) -> Mux1/4, tyre_forces/1(alpha)  "alpha"
  delta/1 -> slip_angles/2(delta), tyre_forces/2(delta)
  eq_of_motion/2(dx_dy_dpsi) -> Mux1/6, slip_angles/1(dx_dy_dpsi)  "dx_dy_dpsi"
  Saturation/1 -> eq_of_motion/1(Vx)

== system Demo_CooperativeDriving_cs/Toyota_Yaris_1/Swarm Behavior/xyalpha_2_state ==
  xyyaw : Inport
  Constant : Constant  Value=0
  Demux : Demux  Outputs=3
  Derivative : Derivative
  Derivative1 : Derivative
  Mux : Mux  Inputs=9
  state : Outport
  wires:
  Demux/1 -> Mux/1, Derivative/1  "x"
  Demux/2 -> Mux/2, Derivative1/1  "y"
  Constant/1 -> Mux/8, Mux/6, Mux/3, Mux/7
  xyyaw/1 -> Demux/1
  Mux/1 -> state/1
  Derivative/1 -> Mux/4
  Derivative1/1 -> Mux/5
  Demux/3 -> Mux/9  "yaw"

== system Demo_CooperativeDriving_cs/BMW_X5_1/SELF_Demux/compas converter/cart2compas ==
  Angle [deg] : Inport
  Constant : Constant  Value=90
  Constant1 : Constant  Value=360
  Gain : Gain  Gain=1/360
  Gain1 : Gain  Gain=360
  Gain2 : Gain  Gain=-1
  Rounding Function : Rounding
  Sum : Sum  Inputs=|-+
  Sum1 : Sum  Inputs=-+|
  Sum2 : Sum  Inputs=++|
  heading [deg] : Outport
  wires:
  Sum2/1 -> heading [deg]/1
  Constant1/1 -> Sum2/1
  Gain2/1 -> Sum2/2
  Constant/1 -> Sum1/1
  Sum1/1 -> Sum/2, Gain/1
  Sum/1 -> Gain2/1
  Angle [deg]/1 -> Sum1/2
  Gain1/1 -> Sum/1
  Rounding Function/1 -> Gain1/1
  Gain/1 -> Rounding Function/1

== system Demo_CooperativeDriving_cs/BMW_X5_1/Swarm Behavior/Vehicle Dynamics/eq_of_motion ==
  Vx : Inport
  F_lat : Inport  Port=2
  Mz : Inport  Port=3
  Fcn1 : Fcn  Expr=u(1)*u(3)
  Gain : Gain  Gain=1/m  SaturateOnIntegerOverflow=on  OutDataTypeStr=Inherit: Same as input  ParamDataTypeStr=Inherit: Same as input
  Gain1 : Gain  Gain=1/Jzz  SaturateOnIntegerOverflow=on  OutDataTypeStr=Inherit: Same as input  ParamDataTypeStr=Inherit: Same as input
  Integrator1 : Integrator
  Integrator4 : Integrator
  Integrator5 : Integrator
  Psip : Integrator
  Sum1 : Sum  Inputs=-+  SaturateOnIntegerOverflow=on  InputSameDT=on  OutDataTypeStr=Inherit: Same as first input
  Vx0 : Fcn  Expr=u(1)*cos(u(3)) - u(2)*sin(u(3))
  "Vy " : Integrator
  Vy0 : Fcn  Expr=u(1)*sin(u(3)) + u(2)*cos(u(3))
  X3 : Mux  Inputs=3
  Xp : Mux  Inputs=3
  Xp1 : Mux  Inputs=2
  Xp2 : Mux  Inputs=3
  x_y_psi : Outport  InitialOutput=0
  dx_dy_dpsi : Outport  Port=2  InitialOutput=0
  ddy_ddpsi : Outport  Port=3  InitialOutput=0
  wires:
  Integrator1/1 -> X3/3, Xp2/3  "psi"
  X3/1 -> x_y_psi/1
  Integrator4/1 -> X3/1  "x"
  Integrator5/1 -> X3/2  "y"
  Vy0/1 -> Integrator5/1
  Vx0/1 -> Integrator4/1
  Xp2/1 -> Vy0/1, Vx0/1
  Mz/1 -> Gain1/1
  Xp1/1 -> ddy_ddpsi/1
  F_lat/1 -> Gain/1
  Sum1/1 -> Xp1/1, "Vy "/1  "dd_y"
  Fcn1/1 -> Sum1/1
  Xp/1 -> dx_dy_dpsi/1, Fcn1/1
  Gain1/1 -> Xp1/2, Psip/1  "dd_psi"
  Vx/1 -> Xp2/1, Xp/1
  Gain/1 -> Sum1/2
  "Vy "/1 -> Xp2/2, Xp/2  "d_y"
  Psip/1 -> Integrator1/1, Xp/3  "d_psi"

== system Demo_CooperativeDriving_cs/BMW_X5_1/Swarm Behavior/Vehicle Dynamics/slip_angles ==
  note: relax_on
      | ON: 1
      | OFF: 0
  dx_dy_dpsi : Inport
  delta : Inport  Port=2
  Constant : Constant  Value=relax_on
  Constant1 : Constant  Value=relax_on
  Mux2 : Mux  Inputs=2
  Sum : Sum  Inputs=++|  SaturateOnIntegerOverflow=on  InputSameDT=on  OutDataTypeStr=Inherit: Same as first input
  Switch : Switch  Threshold=0.5  SaturateOnIntegerOverflow=on  InputSameDT=on
  Switch1 : Switch  Threshold=0.5  SaturateOnIntegerOverflow=on  InputSameDT=on
  alpha_front : Fcn  Expr=-atan( (u(2)+u(3)*lva)/u(1) )
  alpha_rear : Fcn  Expr=-atan( (u(2)-u(3)*laa)/u(1) )
  relaxation_length_front : Subsystem
  relaxation_length_rear : Subsystem
  alpha : Outport
  wires:
  Constant/1 -> Switch/2
  Constant1/1 -> Switch1/2
  Switch1/1 -> Mux2/2  "alpha_r"
  Switch/1 -> Mux2/1  "alpha_f"
  relaxation_length_rear/1(alpha_relax) -> Switch1/1
  relaxation_length_front/1(alpha_relax) -> Switch/1
  alpha_rear/1 -> Switch1/3, relaxation_length_rear/1(alpha_stat)  "alpha_stat_r"
  Sum/1 -> Switch/3, relaxation_length_front/1(alpha_stat)  "alpha_stat_f"
  Mux2/1 -> alpha/1
  dx_dy_dpsi/1 -> relaxation_length_rear/2(dx,dy,dphi), alpha_rear/1, relaxation_length_front/2(dx,dy,dphi), alpha_front/1
  delta/1 -> Sum/1
  alpha_front/1 -> Sum/2

== system Demo_CooperativeDriving_cs/BMW_X5_1/Swarm Behavior/Vehicle Dynamics/tyre_forces ==
  alpha : Inport
  delta : Inport  Port=2
  Demux1 : Demux  Outputs=2
  Fy : Fcn  Expr=u(2)*cos(u(1)) + u(3)
  M2 : Fcn  Expr=u(2)*lva*cos(u(1)) - u(3)*laa
  Mux : Mux  Inputs=2
  Mux2 : Mux  Inputs=3
  tyre_front : Subsystem
  tyre_rear : Subsystem
  Fy_wheels : Outport  InitialOutput=0
  F_lat : Outport  Port=2  InitialOutput=0
  Mz : Outport  Port=3  InitialOutput=0
  wires:
  delta/1 -> Mux2/1
  tyre_rear/1(Fy_r) -> Mux/2, Mux2/3  "Fy_r"
  tyre_front/1(Fy_f) -> Mux/1, Mux2/2  "Fy_f"
  Demux1/2 -> tyre_rear/1(alpha)
  Demux1/1 -> tyre_front/1(alpha)
  alpha/1 -> Demux1/1
  Mux2/1 -> Fy/1, M2/1
  Fy/1 -> F_lat/1
  M2/1 -> Mz/1
  Mux/1 -> Fy_wheels/1

== system Demo_CooperativeDriving_cs/Citroen_C3_1/SELF_Demux/compas converter/cart2compas ==
  Angle [deg] : Inport
  Constant : Constant  Value=90
  Constant1 : Constant  Value=360
  Gain : Gain  Gain=1/360
  Gain1 : Gain  Gain=360
  Gain2 : Gain  Gain=-1
  Rounding Function : Rounding
  Sum : Sum  Inputs=|-+
  Sum1 : Sum  Inputs=-+|
  Sum2 : Sum  Inputs=++|
  heading [deg] : Outport
  wires:
  Sum2/1 -> heading [deg]/1
  Constant1/1 -> Sum2/1
  Gain2/1 -> Sum2/2
  Constant/1 -> Sum1/1
  Sum1/1 -> Sum/2, Gain/1
  Sum/1 -> Gain2/1
  Angle [deg]/1 -> Sum1/2
  Gain1/1 -> Sum/1
  Rounding Function/1 -> Gain1/1
  Gain/1 -> Rounding Function/1

== system Demo_CooperativeDriving_cs/Citroen_C3_1/Swarm Behavior/Vehicle Dynamics/eq_of_motion ==
  Vx : Inport
  F_lat : Inport  Port=2
  Mz : Inport  Port=3
  Fcn1 : Fcn  Expr=u(1)*u(3)
  Gain : Gain  Gain=1/m  SaturateOnIntegerOverflow=on  OutDataTypeStr=Inherit: Same as input  ParamDataTypeStr=Inherit: Same as input
  Gain1 : Gain  Gain=1/Jzz  SaturateOnIntegerOverflow=on  OutDataTypeStr=Inherit: Same as input  ParamDataTypeStr=Inherit: Same as input
  Integrator1 : Integrator
  Integrator4 : Integrator
  Integrator5 : Integrator
  Psip : Integrator
  Sum1 : Sum  Inputs=-+  SaturateOnIntegerOverflow=on  InputSameDT=on  OutDataTypeStr=Inherit: Same as first input
  Vx0 : Fcn  Expr=u(1)*cos(u(3)) - u(2)*sin(u(3))
  "Vy " : Integrator
  Vy0 : Fcn  Expr=u(1)*sin(u(3)) + u(2)*cos(u(3))
  X3 : Mux  Inputs=3
  Xp : Mux  Inputs=3
  Xp1 : Mux  Inputs=2
  Xp2 : Mux  Inputs=3
  x_y_psi : Outport  InitialOutput=0
  dx_dy_dpsi : Outport  Port=2  InitialOutput=0
  ddy_ddpsi : Outport  Port=3  InitialOutput=0
  wires:
  Integrator1/1 -> X3/3, Xp2/3  "psi"
  X3/1 -> x_y_psi/1
  Integrator4/1 -> X3/1  "x"
  Integrator5/1 -> X3/2  "y"
  Vy0/1 -> Integrator5/1
  Vx0/1 -> Integrator4/1
  Xp2/1 -> Vy0/1, Vx0/1
  Mz/1 -> Gain1/1
  Xp1/1 -> ddy_ddpsi/1
  F_lat/1 -> Gain/1
  Sum1/1 -> Xp1/1, "Vy "/1  "dd_y"
  Fcn1/1 -> Sum1/1
  Xp/1 -> dx_dy_dpsi/1, Fcn1/1
  Gain1/1 -> Xp1/2, Psip/1  "dd_psi"
  Vx/1 -> Xp2/1, Xp/1
  Gain/1 -> Sum1/2
  "Vy "/1 -> Xp2/2, Xp/2  "d_y"
  Psip/1 -> Integrator1/1, Xp/3  "d_psi"
